simulink model "mavsim_ue"  (R2021b)
settings: Solver=VariableStepAuto  StartTime=0.0  StopTime=48  RelTol=1e-3  EnableMultiTasking=on
InitFcn:
  | param_quad
undefined symbols (not defined in the file or in its folder): P
libraries: slpidlib x4, simulink x1, visionsinks x1, sim3dcameralib x1, sim3dlib x1, uavsim3dlib x1
settings Model: PauseTimes=0.1  Creator=beard  LastModifiedBy=brian
settings SolverCC: ZeroCrossAlgorithm=Adaptive  AlgebraicLoopSolver=TrustRegion
settings DataIOCC: LimitDataPoints=on  SaveFormat=Array  ReturnWorkspaceOutputs=off
settings OptimizationCC: ExpressionDepthLimit=2147483647  InitFltsAndDblsToZero=on  LifeSpan=inf
settings DebuggingCC: UnderspecifiedInitializationDetection=Classic  MergeDetectMultiDrivingBlocksExec=none  IgnoredZcDiagnostic=none  SolverPrmCheckMsg=warning  MultiTaskDSMMsg=warning  MultiTaskCondExecSysMsg=none  StateNameClashWarn=warning  SFUnexpectedBacktrackingDiag=warning  SFNoUnconditionalDefaultTransitionDiag=warning  SFExecutionAtInitializationDiag=none  SFMachineParentedDataDiag=warning  ArithmeticOperatorsInVariantConditions=warning
settings HardwareCC: ProdBitPerPointer=32  ProdBitPerSizeT=32  ProdBitPerPtrDiffT=32  ProdLargestAtomicFloat=None  ProdIntDivRoundTo=Undefined  ProdEndianess=Unspecified  ProdWordSize=32  ProdHWDeviceType=32-bit Generic
settings ModelReferenceCC: PropagateSignalLabelsOutOfModel=off
settings SFSimCC: SimUseLocalCustomCode=off  CustomCodeUndefinedFunction=UseInterfaceOnly
settings RTWCC: RTWUseLocalCustomCode=off
settings CodeAppCC: StateflowObjectComments=on
settings GRTTargetCC: TargetLangStandard=C89/C90 (ANSI)  CombineOutputUpdateFcns=off  GRTInterface=on
settings ConfigComp: CovMetricSettings=dw  CovSaveCumulativeToWorkspaceVar=on  CovSaveSingleToWorkspaceVar=on  CovExternalEMLEnable=off  CovSFcnEnable=off

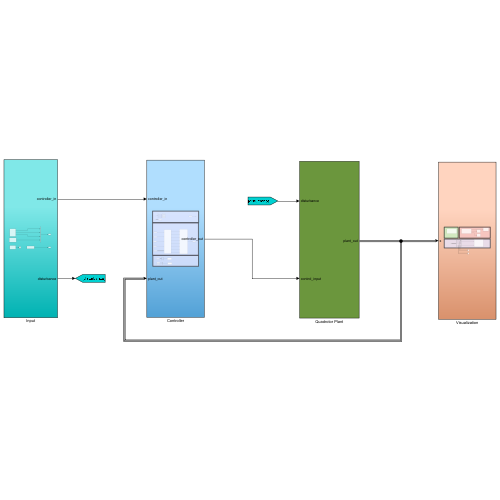
[thumbnail: Simulink's stored preview of the top-level diagram]
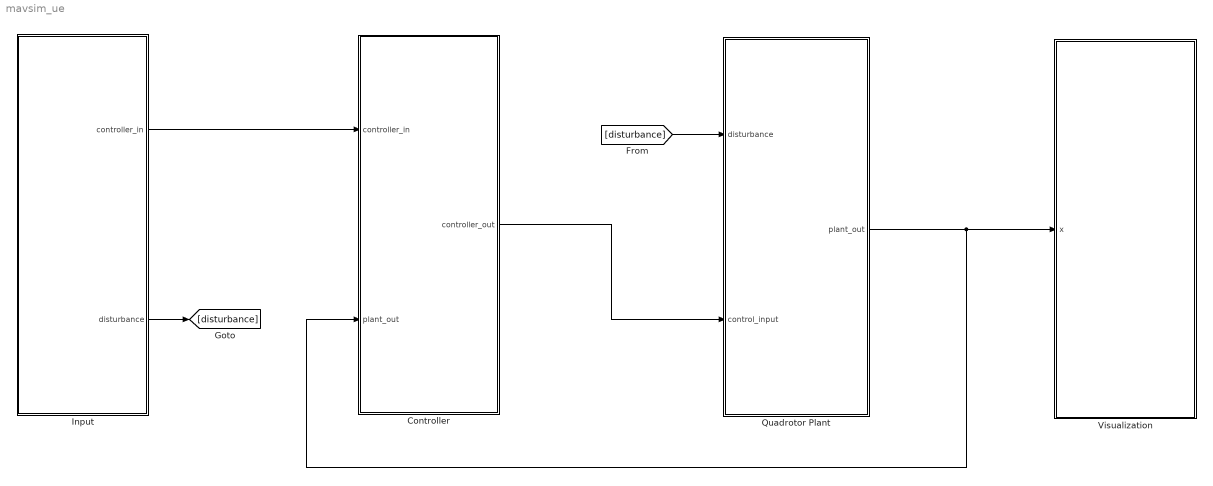
== system mavsim_ue ==
  Controller : Subsystem
  Input : Subsystem
  Quadrotor Plant : Subsystem
  Visualization : Subsystem
  wires:
  Input/2(disturbance) -> [disturbance]
  [disturbance] -> Quadrotor Plant/1(disturbance)
  Quadrotor Plant/1(plant_out) -> Visualization/1(x), Controller/2(plant_out)
  Controller/1(controller_out) -> Quadrotor Plant/2(control_input)
  Input/1(controller_in) -> Controller/1(controller_in)

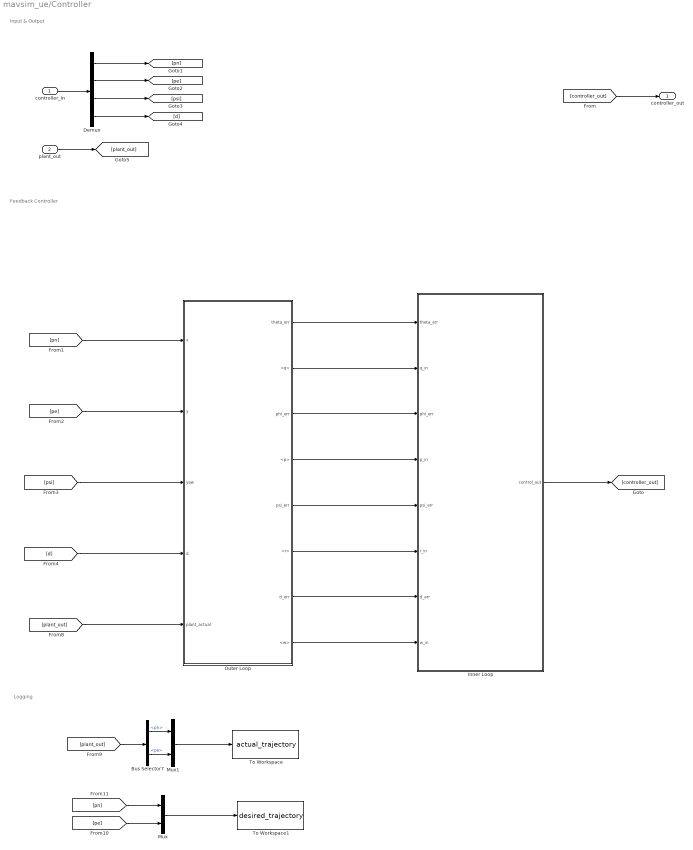
== system mavsim_ue/Controller ==
  note: Logging
  note: Input & Output
  note: Feedback Controller
  controller_in : Inport
  plant_out : Inport  Port=2
  Bus Selector7 : BusSelector  OutputSignals=pn,pe
  Demux : Demux
  Inner Loop : Subsystem
  Mux : Mux  Inputs=2
  Mux1 : Mux  Inputs=2
  Outer Loop : Subsystem
  To Workspace : ToWorkspace  VariableName=actual_trajectory  SaveFormat=Timeseries  SampleTime=-1
  To Workspace1 : ToWorkspace  VariableName=desired_trajectory  SaveFormat=Timeseries  SampleTime=-1
  controller_out : Outport  VectorParamsAs1DForOutWhenUnconnected=off
  wires:
  Inner Loop/1(control_out) -> [controller_out]
  [controller_out] -> controller_out/1
  Demux/1 -> [pn]
  Demux/2 -> [pe]
  Demux/3 -> [psi]
  Demux/4 -> [d]
  plant_out/1 -> [plant_out]
  controller_in/1 -> Demux/1
  [plant_out] -> Bus Selector7/1
  [pe] -> Mux/2
  [pn] -> Mux/1
  Bus Selector7/2 -> Mux1/2  "<pe>"
  Bus Selector7/1 -> Mux1/1  "<pn>"
  Mux1/1 -> To Workspace/1
  Mux/1 -> To Workspace1/1
  [pn] -> Outer Loop/1(x)
  [plant_out] -> Outer Loop/5(plant_actual)
  [pe] -> Outer Loop/2(y)
  [psi] -> Outer Loop/3(yaw)
  [d] -> Outer Loop/4(d)
  Outer Loop/1(theta_err) -> Inner Loop/1(theta_err)
  Outer Loop/2(<q>) -> Inner Loop/2(q_in)
  Outer Loop/3(phi_err) -> Inner Loop/3(phi_err)
  Outer Loop/4(<p>) -> Inner Loop/4(p_in)
  Outer Loop/5(psi_err) -> Inner Loop/5(psi_err)
  Outer Loop/6(<r>) -> Inner Loop/6(r_in)
  Outer Loop/7(d_err) -> Inner Loop/7(d_err)
  Outer Loop/8(<w>) -> Inner Loop/8(w_in)

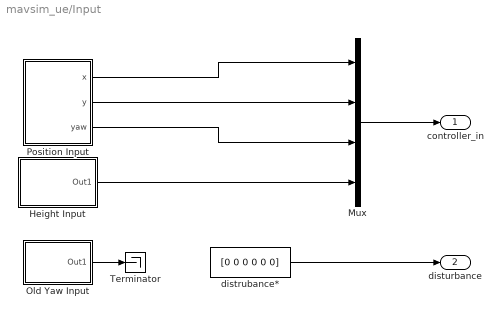
== system mavsim_ue/Input ==
  Height Input : Subsystem
  Mux : Mux
  Old Yaw Input : Subsystem
  Position Input : Subsystem
  Terminator : Terminator
  distrubance* : Constant  Value=[0 0 0 0 0 0]  SampleTime=0
  controller_in : Outport  VectorParamsAs1DForOutWhenUnconnected=off
  disturbance : Outport  Port=2  VectorParamsAs1DForOutWhenUnconnected=off
  wires:
  distrubance*/1 -> disturbance/1
  Mux/1 -> controller_in/1
  Position Input/1(x) -> Mux/1
  Position Input/2(y) -> Mux/2
  Old Yaw Input/1(Out1) -> Terminator/1
  Height Input/1(Out1) -> Mux/4
  Position Input/3(yaw) -> Mux/3

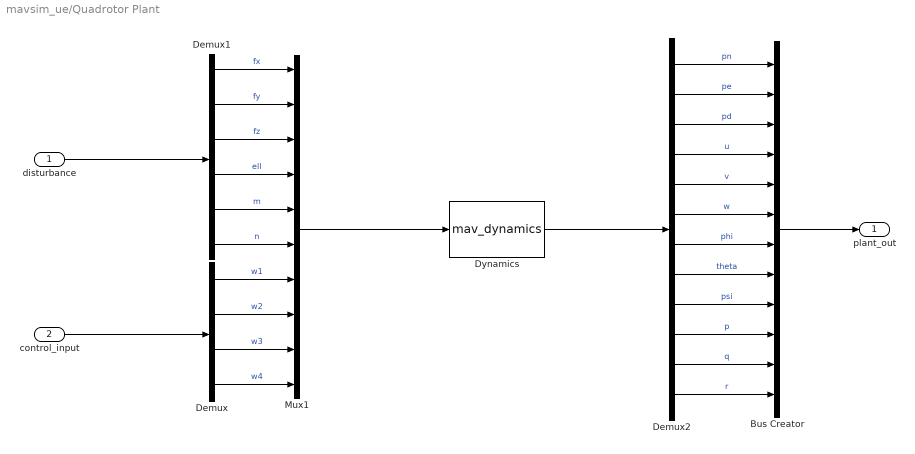
== system mavsim_ue/Quadrotor Plant ==
  disturbance : Inport
  control_input : Inport  Port=2
  Bus Creator : BusCreator  Inputs=12
  Demux : Demux
  Demux1 : Demux  Outputs=6
  Demux2 : Demux  Outputs=12
  Dynamics : S-Function  FunctionName=mav_dynamics  Parameters=P  SFunctionDeploymentMode=off  EnableBusSupport=off
  Mux1 : Mux  Inputs=10
  plant_out : Outport  VectorParamsAs1DForOutWhenUnconnected=off
  wires:
  Dynamics/1 -> Demux2/1
  Demux2/12 -> Bus Creator/12  "r"
  Demux2/1 -> Bus Creator/1  "pn"
  Demux2/2 -> Bus Creator/2  "pe"
  Demux2/3 -> Bus Creator/3  "pd"
  Demux2/4 -> Bus Creator/4  "u"
  Demux2/5 -> Bus Creator/5  "v"
  Demux2/6 -> Bus Creator/6  "w"
  Demux2/8 -> Bus Creator/8  "theta"
  Demux2/7 -> Bus Creator/7  "phi"
  Demux2/9 -> Bus Creator/9  "psi"
  Demux2/10 -> Bus Creator/10  "p"
  Demux2/11 -> Bus Creator/11  "q"
  control_input/1 -> Demux/1
  Bus Creator/1 -> plant_out/1
  Mux1/1 -> Dynamics/1
  Demux/2 -> Mux1/8  "w2"
  Demux1/5 -> Mux1/5  "m"
  Demux1/4 -> Mux1/4  "ell"
  Demux/4 -> Mux1/10  "w4"
  Demux/1 -> Mux1/7  "w1"
  Demux1/6 -> Mux1/6  "n"
  Demux1/2 -> Mux1/2  "fy"
  Demux1/3 -> Mux1/3  "fz"
  Demux/3 -> Mux1/9  "w3"
  Demux1/1 -> Mux1/1  "fx"
  disturbance/1 -> Demux1/1

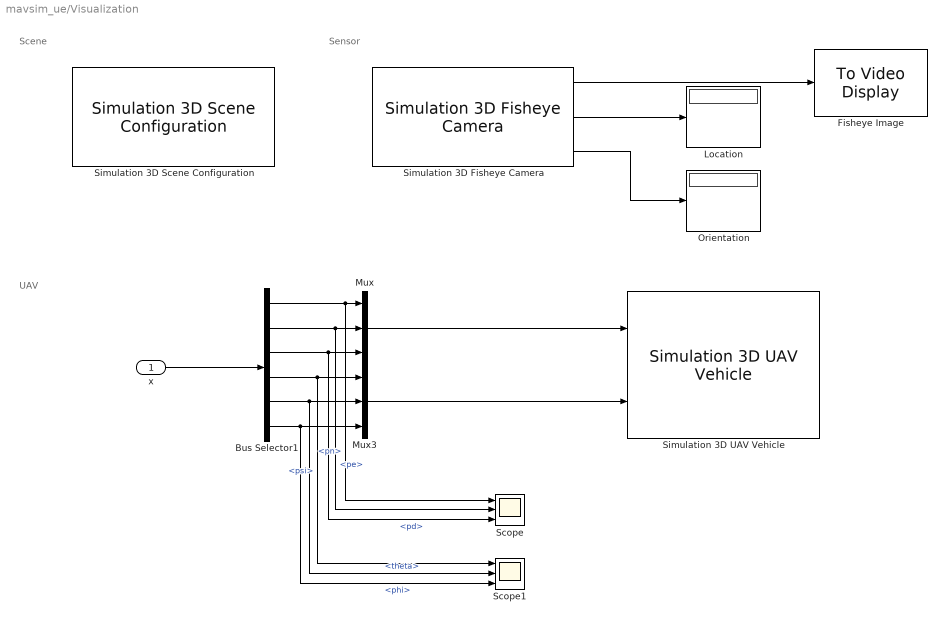
== system mavsim_ue/Visualization ==
  note: Sensor
  note: UAV
  note: Scene
  x : Inport
  Bus Selector1 : BusSelector  OutputSignals=pn,pe,pd,psi,theta,phi
  Fisheye Image : visionsinks/To Video Display  windowSizeMode=Normal  openAtMdlStart=on  fullScreen=off  videoWindowX=3199  videoWindowY=680  saveWindowSize=off  videoWindowWidth=640  videoWindowHeight=502  inputColorFormat=RGB  inputType=Obsolete  imagePorts=One multidimensional signal  OutputDevice=On-screen video monitor  dataOrg=Column-major  isWindowOpen=off
  Location : Display
  Mux : Mux  Inputs=3
  Mux3 : Mux  Inputs=3
  Orientation : Display
  Scope : Scope  NumInputPorts=3
  Scope1 : Scope  NumInputPorts=3
  Simulation 3D Fisheye Camera : sim3dcameralib/Simulation 3D Fisheye Camera  Priority=1  sensorTag=Sim3dSensor2  sensorId=2  sensorName=Sim3dSensor2  vehTagList={'Scene Origin';'SimulinkVehicle2'}  vehTag=SimulinkVehicle2  mountLoc=Origin  offsetFlag=on  tmountOffset=[0.1, 0, 0]  extTmount=off  rmountOffset=[0, 0, 0]  extRmount=off  OpticalCenter=[640, 360]  ImageSize=[720, 1280]  RadialDistortion=[320, -0.0005, 0, 0]  StretchMatrix=[1, 0; 0, 1]  TransformOutportEnabled=on  SampleTime=-1  mountPoint=[0.1 0 0]  mountOrientation=[0 0 0]  aMode=4  ID=2
      settings: SourceProductBaseCode=AE,DR,UV,VE
  Simulation 3D Scene Configuration : sim3dlib/Simulation 3D Scene Configuration  Priority=0  ProjectFormat_internal=Default Scenes  ProjectFormat=Default Scenes  SceneDesc=US city block  ProjectName=C:\Program Files\MATLAB\R2021b\toolbox\shared\sim3d_projects\automotive_project\UE4\WindowsNoEditor\VehicleSimulation.exe  ScenePath=/Game/Maps/USCityBlock  vehTagList={'Scene Origin';'SimulinkVehicle2'}  vehTag=SimulinkVehicle2  OpVisEn=off  Ts=1/60  EnableWindow=on  EnableWeather=off  SunAltitude=40.0  SunAzimuth=90  clouds=10  wind=1  fog=0  rain=0  sensorTag=MainCamera2  sensorId=2  sensorName=MainCamera2  mountLoc=Origin  offsetFlag=off  tmountOffset=[0, 0, 0]  rmountOffset=[0, 0, 0]  HorizontalResolution=1280  VerticalResolution=720  HorizontalFOV=60  mountPoint=[0 0 0]  mountOrientation=[0 0 0]  aMode=4  ID=2
      settings: SourceProductBaseCode=AE,DR,UV,VE
  Simulation 3D UAV Vehicle : uavsim3dlib/Simulation 3D UAV Vehicle  Mesh=Quadrotor  MeshPath=/MathWorksUAVContent/UAVs/HexaRotorUAV/HexaRotor.HexaRotor  Color=Orange  ActorName=SimulinkVehicle2  InitialTranslation=[0 5 1.5]  InitialRotation=[0 0 0]  SampleTime=-1  ActorType=SimulinkVehicle  ID=2  aMode=4  ActorTag=SimulinkVehicle2
      settings: SourceProductBaseCode=UV
  wires:
  Bus Selector1/2 -> Scope/2, Mux/2  "<pe>"
  Simulation 3D Fisheye Camera/3 -> Orientation/1
  Bus Selector1/6 -> Scope1/3, Mux3/3  "<phi>"
  Simulation 3D Fisheye Camera/1 -> Fisheye Image/1
  Bus Selector1/5 -> Scope1/2, Mux3/2  "<theta>"
  Simulation 3D Fisheye Camera/2 -> Location/1
  x/1 -> Bus Selector1/1
  Mux3/1 -> Simulation 3D UAV Vehicle/2
  Mux/1 -> Simulation 3D UAV Vehicle/1
  Bus Selector1/1 -> Scope/1, Mux/1  "<pn>"
  Bus Selector1/3 -> Scope/3, Mux/3  "<pd>"
  Bus Selector1/4 -> Scope1/1, Mux3/1  "<psi>"

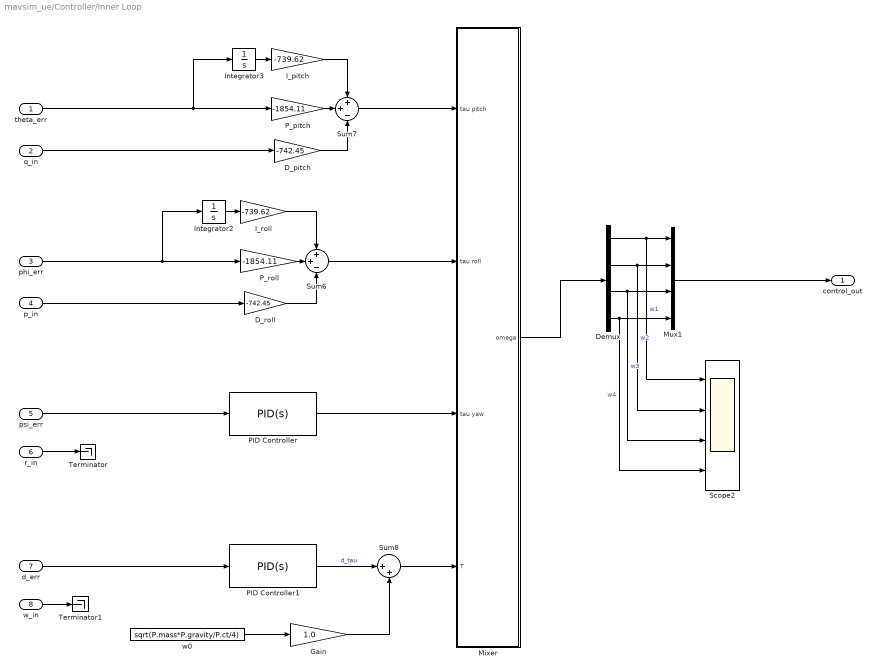
== system mavsim_ue/Controller/Inner Loop ==
  theta_err : Inport
  q_in : Inport  Port=2
  phi_err : Inport  Port=3
  p_in : Inport  Port=4
  psi_err : Inport  Port=5
  r_in : Inport  Port=6
  d_err : Inport  Port=7
  w_in : Inport  Port=8
  D_pitch : Gain  Gain=-742.45
  D_roll : Gain  Gain=-742.45
  Demux : Demux
  Gain : Gain  Gain=1.0
  I_pitch : Gain  Gain=-739.62
  I_roll : Gain  Gain=-739.62
  Integrator2 : Integrator
  Integrator3 : Integrator
  Mixer : Subsystem
  Mux1 : Mux
  PID Controller : slpidlib/PID Controller  Controller=PID  Form=Parallel  TimeDomain=Continuous-time  UseExternalTs=off  SampleTime=1  IntegratorMethod=Forward Euler  FilterMethod=Forward Euler  ControllerParametersSource=internal  P=-13367.2156192971  I=-5976.18350297239  D=-7341.77839074489  UseFilter=on  N=52.0850115715791  TunerSelectOption=Transfer Function Based (PID Tuner App)  InitialConditionSource=internal  InitialConditionForIntegrator=0  InitialConditionForFilter=0  DifferentiatorICPrevScaledInput=0  ExternalReset=none  TrackingMode=off  Kt=1  LimitOutput=off  SatLimitsSource=internal  UpperSaturationLimit=pi/3  LowerSaturationLimit=-pi/3  LinearizeAsGain=off  AntiWindupMode=clamping  Kb=1.5  POutMin=[]  POutMax=[]  IOutMin=[]  IOutMax=[]  DOutMin=[]  DOutMax=[]  NOutMin=[]  NOutMax=[]  SumOutMin=[]  SumOutMax=[]  SaturationOutMin=[]  SaturationOutMax=[]  PParamMin=[]  PParamMax=[]  IParamMin=[]  IParamMax=[]  DParamMin=[]  DParamMax=[]  NParamMin=[]  NParamMax=[]  KbParamMin=[]  KbParamMax=[]  KtParamMin=[]  KtParamMax=[]  KbOutMin=[]  KbOutMax=[]  KtOutMin=[]  KtOutMax=[]  IntegratorOutMin=[]  IntegratorOutMax=[]  FilterOutMin=[]  FilterOutMax=[]  SumI1OutMin=[]  SumI1OutMax=[]  SumI2OutMin=[]  SumI2OutMax=[]  SumI3OutMin=[]  SumI3OutMax=[]  SumI4OutMin=[]  SumI4OutMax=[]  SumDOutMin=[]  SumDOutMax=[]  DifferentiatorOutMin=[]  DifferentiatorOutMax=[]  FilterDiffOutCoefMin=[]  FilterDiffOutCoefMax=[]  ReciprocalOutMin=[]  ReciprocalOutMax=[]  SumDenOutMin=[]  SumDenOutMax=[]  SumNumOutMin=[]  SumNumOutMax=[]  DivideOutMin=[]  DivideOutMax=[]  UdiffTsProdOutMin=[]  UdiffTsProdOutMax=[]  NTsProdOutMin=[]  NTsProdOutMax=[]  UintegralTsProdOutMin=[]  UintegralTsProdOutMax=[]  UngainTsProdOutMin=[]  UngainTsProdOutMax=[]  IntegratorContinuousStateAttributes=''  IntegratorStateMustResolveToSignalObject=off  IntegratorRTWStateStorageClass=Auto  FilterContinuousStateAttributes=''  FilterStateMustResolveToSignalObject=off  FilterRTWStateStorageClass=Auto  ParallelPVariant=InternalParameters  IdealPVariant=Disabled  IVariant=InternalParameters  DVariant=InternalParameters  IntegratorVariant=Continuous  SatVariant=Disabled  AWVariant=Passthrough  PCopyVariant=Disabled  TRVariant=Disabled  FdbkBlocksVariant=Forward  IdealPFdbkVariant=Disabled  SatFdbkVariant=Disabled  DerivativeFilterVariant=ContFilter  NVariant=InternalParameters  NCopyVariant=Disabled  FilterICVariant=InternalICsFilter  IntegratorICVariant=InternalICs  ExternalResetVariant=Disabled  TRSumVariant=Passthrough  SumFdbkVariant=Disabled  SumVariant=Sum_PID  TsampFilterVariant=InternalTs  TsampNgainVariant=Passthrough  TsampIntegralVariant=Passthrough  ExternalSaturationOutDataTypeStr=Inherit: Same as second input
  PID Controller1 : slpidlib/PID Controller  Controller=PID  Form=Parallel  TimeDomain=Continuous-time  UseExternalTs=off  SampleTime=1  IntegratorMethod=Forward Euler  FilterMethod=Forward Euler  ControllerParametersSource=internal  P=949.514869239601  I=444.513280768002  D=498.037549912903  UseFilter=on  N=54.5397025421619  TunerSelectOption=Transfer Function Based (PID Tuner App)  InitialConditionSource=internal  InitialConditionForIntegrator=0  InitialConditionForFilter=0  DifferentiatorICPrevScaledInput=0  ExternalReset=none  TrackingMode=off  Kt=1  LimitOutput=off  SatLimitsSource=internal  UpperSaturationLimit=pi/3  LowerSaturationLimit=-pi/3  LinearizeAsGain=off  AntiWindupMode=clamping  Kb=1.5  POutMin=[]  POutMax=[]  IOutMin=[]  IOutMax=[]  DOutMin=[]  DOutMax=[]  NOutMin=[]  NOutMax=[]  SumOutMin=[]  SumOutMax=[]  SaturationOutMin=[]  SaturationOutMax=[]  PParamMin=[]  PParamMax=[]  IParamMin=[]  IParamMax=[]  DParamMin=[]  DParamMax=[]  NParamMin=[]  NParamMax=[]  KbParamMin=[]  KbParamMax=[]  KtParamMin=[]  KtParamMax=[]  KbOutMin=[]  KbOutMax=[]  KtOutMin=[]  KtOutMax=[]  IntegratorOutMin=[]  IntegratorOutMax=[]  FilterOutMin=[]  FilterOutMax=[]  SumI1OutMin=[]  SumI1OutMax=[]  SumI2OutMin=[]  SumI2OutMax=[]  SumI3OutMin=[]  SumI3OutMax=[]  SumI4OutMin=[]  SumI4OutMax=[]  SumDOutMin=[]  SumDOutMax=[]  DifferentiatorOutMin=[]  DifferentiatorOutMax=[]  FilterDiffOutCoefMin=[]  FilterDiffOutCoefMax=[]  ReciprocalOutMin=[]  ReciprocalOutMax=[]  SumDenOutMin=[]  SumDenOutMax=[]  SumNumOutMin=[]  SumNumOutMax=[]  DivideOutMin=[]  DivideOutMax=[]  UdiffTsProdOutMin=[]  UdiffTsProdOutMax=[]  NTsProdOutMin=[]  NTsProdOutMax=[]  UintegralTsProdOutMin=[]  UintegralTsProdOutMax=[]  UngainTsProdOutMin=[]  UngainTsProdOutMax=[]  IntegratorContinuousStateAttributes=''  IntegratorStateMustResolveToSignalObject=off  IntegratorRTWStateStorageClass=Auto  FilterContinuousStateAttributes=''  FilterStateMustResolveToSignalObject=off  FilterRTWStateStorageClass=Auto  ParallelPVariant=InternalParameters  IdealPVariant=Disabled  IVariant=InternalParameters  DVariant=InternalParameters  IntegratorVariant=Continuous  SatVariant=Disabled  AWVariant=Passthrough  PCopyVariant=Disabled  TRVariant=Disabled  FdbkBlocksVariant=Forward  IdealPFdbkVariant=Disabled  SatFdbkVariant=Disabled  DerivativeFilterVariant=ContFilter  NVariant=InternalParameters  NCopyVariant=Disabled  FilterICVariant=InternalICsFilter  IntegratorICVariant=InternalICs  ExternalResetVariant=Disabled  TRSumVariant=Passthrough  SumFdbkVariant=Disabled  SumVariant=Sum_PID  TsampFilterVariant=InternalTs  TsampNgainVariant=Passthrough  TsampIntegralVariant=Passthrough  ExternalSaturationOutDataTypeStr=Inherit: Same as second input
  P_pitch : Gain  Gain=-1854.11
  P_roll : Gain  Gain=-1854.11
  Scope2 : Scope  NumInputPorts=4
  Sum6 : Sum  Inputs=++-
  Sum7 : Sum  Inputs=++-
  Sum8 : Sum  Inputs=|++
  Terminator : Terminator
  Terminator1 : Terminator
  w0 : Constant  Value=sqrt(P.mass*P.gravity/P.ct/4)  SampleTime=0
  control_out : Outport  VectorParamsAs1DForOutWhenUnconnected=off
  wires:
  r_in/1 -> Terminator/1
  P_pitch/1 -> Sum7/2
  P_roll/1 -> Sum6/2
  Demux/4 -> Mux1/4, Scope2/4  "w4"
  Demux/1 -> Mux1/1, Scope2/1  "w1"
  theta_err/1 -> Integrator3/1, P_pitch/1
  Demux/2 -> Mux1/2, Scope2/2  "w2"
  Sum8/1 -> Mixer/4(T)
  Mixer/1(omega) -> Demux/1
  phi_err/1 -> Integrator2/1, P_roll/1
  D_roll/1 -> Sum6/3
  Integrator2/1 -> I_roll/1
  Integrator3/1 -> I_pitch/1
  D_pitch/1 -> Sum7/3
  Demux/3 -> Mux1/3, Scope2/3  "w3"
  I_pitch/1 -> Sum7/1
  q_in/1 -> D_pitch/1
  w0/1 -> Gain/1
  I_roll/1 -> Sum6/1
  Mux1/1 -> control_out/1
  Sum6/1 -> Mixer/2(tau roll)
  w_in/1 -> Terminator1/1
  Sum7/1 -> Mixer/1(tau pitch)
  p_in/1 -> D_roll/1
  psi_err/1 -> PID Controller/1
  PID Controller/1 -> Mixer/3(tau yaw)
  PID Controller1/1 -> Sum8/1  "d_tau"
  d_err/1 -> PID Controller1/1
  Gain/1 -> Sum8/2

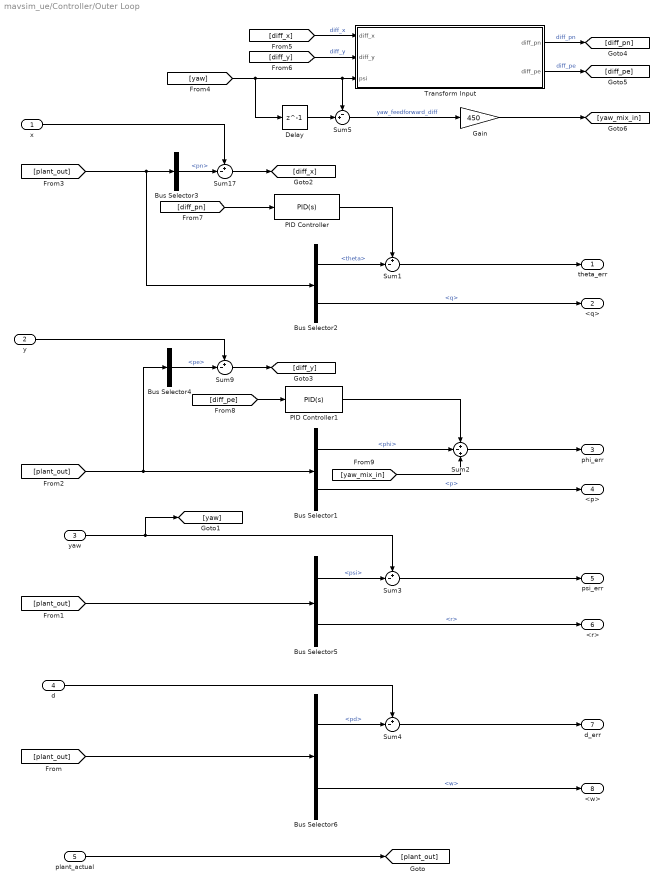
== system mavsim_ue/Controller/Outer Loop ==
  x : Inport
  y : Inport  Port=2
  yaw : Inport  Port=3
  d : Inport  Port=4
  plant_actual : Inport  Port=5
  Bus Selector1 : BusSelector  OutputSignals=phi,p
  Bus Selector2 : BusSelector  OutputSignals=theta,q
  Bus Selector3 : BusSelector  OutputSignals=pn
  Bus Selector4 : BusSelector  OutputSignals=pe
  Bus Selector5 : BusSelector  OutputSignals=psi,r
  Bus Selector6 : BusSelector  OutputSignals=pd,w
  Delay : Delay  DelayLength=1
  Gain : Gain  Gain=450
  PID Controller : slpidlib/PID Controller  Controller=PID  Form=Parallel  TimeDomain=Continuous-time  UseExternalTs=off  SampleTime=1  IntegratorMethod=Forward Euler  FilterMethod=Forward Euler  ControllerParametersSource=internal  P=0.00699656063641612  I=6.00915879281628e-05  D=0.106583930326049  UseFilter=on  N=132.721128235741  TunerSelectOption=Transfer Function Based (PID Tuner App)  InitialConditionSource=internal  InitialConditionForIntegrator=0  InitialConditionForFilter=0  DifferentiatorICPrevScaledInput=0  ExternalReset=none  TrackingMode=off  Kt=0.1  LimitOutput=on  SatLimitsSource=internal  UpperSaturationLimit=pi/2.2  LowerSaturationLimit=-pi/2.2  LinearizeAsGain=off  AntiWindupMode=clamping  Kb=1.5  POutMin=[]  POutMax=[]  IOutMin=[]  IOutMax=[]  DOutMin=[]  DOutMax=[]  NOutMin=[]  NOutMax=[]  SumOutMin=[]  SumOutMax=[]  SaturationOutMin=[]  SaturationOutMax=[]  PParamMin=[]  PParamMax=[]  IParamMin=[]  IParamMax=[]  DParamMin=[]  DParamMax=[]  NParamMin=[]  NParamMax=[]  KbParamMin=[]  KbParamMax=[]  KtParamMin=[]  KtParamMax=[]  KbOutMin=[]  KbOutMax=[]  KtOutMin=[]  KtOutMax=[]  IntegratorOutMin=[]  IntegratorOutMax=[]  FilterOutMin=[]  FilterOutMax=[]  SumI1OutMin=[]  SumI1OutMax=[]  SumI2OutMin=[]  SumI2OutMax=[]  SumI3OutMin=[]  SumI3OutMax=[]  SumI4OutMin=[]  SumI4OutMax=[]  SumDOutMin=[]  SumDOutMax=[]  DifferentiatorOutMin=[]  DifferentiatorOutMax=[]  FilterDiffOutCoefMin=[]  FilterDiffOutCoefMax=[]  ReciprocalOutMin=[]  ReciprocalOutMax=[]  SumDenOutMin=[]  SumDenOutMax=[]  SumNumOutMin=[]  SumNumOutMax=[]  DivideOutMin=[]  DivideOutMax=[]  UdiffTsProdOutMin=[]  UdiffTsProdOutMax=[]  NTsProdOutMin=[]  NTsProdOutMax=[]  UintegralTsProdOutMin=[]  UintegralTsProdOutMax=[]  UngainTsProdOutMin=[]  UngainTsProdOutMax=[]  IntegratorContinuousStateAttributes=''  IntegratorStateMustResolveToSignalObject=off  IntegratorRTWStateStorageClass=Auto  FilterContinuousStateAttributes=''  FilterStateMustResolveToSignalObject=off  FilterRTWStateStorageClass=Auto  ParallelPVariant=InternalParameters  IdealPVariant=Disabled  IVariant=InternalParameters  DVariant=InternalParameters  IntegratorVariant=Continuous  SatVariant=Enabled  AWVariant=ContClampingParallel  PCopyVariant=Disabled  TRVariant=Disabled  FdbkBlocksVariant=Forward  IdealPFdbkVariant=Disabled  SatFdbkVariant=Disabled  DerivativeFilterVariant=ContFilter  NVariant=InternalParameters  NCopyVariant=Disabled  FilterICVariant=InternalICsFilter  IntegratorICVariant=InternalICs  ExternalResetVariant=Disabled  TRSumVariant=Passthrough  SumFdbkVariant=Disabled  SumVariant=Sum_PID  TsampFilterVariant=InternalTs  TsampNgainVariant=Passthrough  TsampIntegralVariant=Passthrough  ExternalSaturationOutDataTypeStr=Inherit: Same as second input
  PID Controller1 : slpidlib/PID Controller  Controller=PID  Form=Parallel  TimeDomain=Continuous-time  UseExternalTs=off  SampleTime=1  IntegratorMethod=Forward Euler  FilterMethod=Forward Euler  ControllerParametersSource=internal  P=-0.0043801368418265  I=-3.38745804747184e-05  D=-0.112019721849609  UseFilter=on  N=138.65464157868  TunerSelectOption=Transfer Function Based (PID Tuner App)  InitialConditionSource=internal  InitialConditionForIntegrator=0  InitialConditionForFilter=0  DifferentiatorICPrevScaledInput=0  ExternalReset=none  TrackingMode=off  Kt=0.75  LimitOutput=on  SatLimitsSource=internal  UpperSaturationLimit=pi/2.2  LowerSaturationLimit=-pi/2.2  LinearizeAsGain=off  AntiWindupMode=clamping  Kb=1  POutMin=[]  POutMax=[]  IOutMin=[]  IOutMax=[]  DOutMin=[]  DOutMax=[]  NOutMin=[]  NOutMax=[]  SumOutMin=[]  SumOutMax=[]  SaturationOutMin=[]  SaturationOutMax=[]  PParamMin=[]  PParamMax=[]  IParamMin=[]  IParamMax=[]  DParamMin=[]  DParamMax=[]  NParamMin=[]  NParamMax=[]  KbParamMin=[]  KbParamMax=[]  KtParamMin=[]  KtParamMax=[]  KbOutMin=[]  KbOutMax=[]  KtOutMin=[]  KtOutMax=[]  IntegratorOutMin=[]  IntegratorOutMax=[]  FilterOutMin=[]  FilterOutMax=[]  SumI1OutMin=[]  SumI1OutMax=[]  SumI2OutMin=[]  SumI2OutMax=[]  SumI3OutMin=[]  SumI3OutMax=[]  SumI4OutMin=[]  SumI4OutMax=[]  SumDOutMin=[]  SumDOutMax=[]  DifferentiatorOutMin=[]  DifferentiatorOutMax=[]  FilterDiffOutCoefMin=[]  FilterDiffOutCoefMax=[]  ReciprocalOutMin=[]  ReciprocalOutMax=[]  SumDenOutMin=[]  SumDenOutMax=[]  SumNumOutMin=[]  SumNumOutMax=[]  DivideOutMin=[]  DivideOutMax=[]  UdiffTsProdOutMin=[]  UdiffTsProdOutMax=[]  NTsProdOutMin=[]  NTsProdOutMax=[]  UintegralTsProdOutMin=[]  UintegralTsProdOutMax=[]  UngainTsProdOutMin=[]  UngainTsProdOutMax=[]  IntegratorContinuousStateAttributes=''  IntegratorStateMustResolveToSignalObject=off  IntegratorRTWStateStorageClass=Auto  FilterContinuousStateAttributes=''  FilterStateMustResolveToSignalObject=off  FilterRTWStateStorageClass=Auto  ParallelPVariant=InternalParameters  IdealPVariant=Disabled  IVariant=InternalParameters  DVariant=InternalParameters  IntegratorVariant=Continuous  SatVariant=Enabled  AWVariant=ContClampingParallel  PCopyVariant=Disabled  TRVariant=Disabled  FdbkBlocksVariant=Forward  IdealPFdbkVariant=Disabled  SatFdbkVariant=Disabled  DerivativeFilterVariant=ContFilter  NVariant=InternalParameters  NCopyVariant=Disabled  FilterICVariant=InternalICsFilter  IntegratorICVariant=InternalICs  ExternalResetVariant=Disabled  TRSumVariant=Passthrough  SumFdbkVariant=Disabled  SumVariant=Sum_PID  TsampFilterVariant=InternalTs  TsampNgainVariant=Passthrough  TsampIntegralVariant=Passthrough  ExternalSaturationOutDataTypeStr=Inherit: Same as second input
  Sum{1,3..4,9,17} (5 alike) : Sum  Inputs=+-|
  Sum2 : Sum  Inputs=+-+
  Sum5 : Sum  Inputs=-+|
  Transform Input : MATLAB Function  TreatAsAtomicUnit=on
  theta_err : Outport
  <q> : Outport  Port=2
  phi_err : Outport  Port=3
  <p> : Outport  Port=4
  psi_err : Outport  Port=5
  <r> : Outport  Port=6
  d_err : Outport  Port=7
  <w> : Outport  Port=8
  wires:
  [plant_out] -> Bus Selector2/1, Bus Selector3/1
  Bus Selector4/1 -> Sum9/2  "<pe>"
  Bus Selector2/1 -> Sum1/2  "<theta>"
  Bus Selector6/2 -> <w>/1  "<w>"
  Bus Selector1/1 -> Sum2/2  "<phi>"
  Bus Selector3/1 -> Sum17/2  "<pn>"
  Bus Selector5/1 -> Sum3/2  "<psi>"
  Bus Selector6/1 -> Sum4/2  "<pd>"
  [plant_out] -> Bus Selector5/1
  Bus Selector2/2 -> <q>/1  "<q>"
  [plant_out] -> Bus Selector4/1, Bus Selector1/1
  Sum9/1 -> [diff_y]
  [plant_out] -> Bus Selector6/1
  yaw/1 -> [yaw], Sum3/1
  x/1 -> Sum17/1
  Sum3/1 -> psi_err/1
  y/1 -> Sum9/1
  Bus Selector5/2 -> <r>/1  "<r>"
  Bus Selector1/2 -> <p>/1  "<p>"
  plant_actual/1 -> [plant_out]
  Sum4/1 -> d_err/1
  d/1 -> Sum4/1
  Sum17/1 -> [diff_x]
  Sum1/1 -> theta_err/1
  Sum2/1 -> phi_err/1
  [yaw] -> Delay/1, Transform Input/3(psi), Sum5/1
  [diff_x] -> Transform Input/1(diff_x)  "diff_x"
  [diff_y] -> Transform Input/2(diff_y)  "diff_y"
  Transform Input/1(diff_pn) -> [diff_pn]  "diff_pn"
  [diff_pn] -> PID Controller/1
  [diff_pe] -> PID Controller1/1
  Delay/1 -> Sum5/2
  Sum5/1 -> Gain/1  "yaw_feedforward_diff"
  Transform Input/2(diff_pe) -> [diff_pe]  "diff_pe"
  Gain/1 -> [yaw_mix_in]
  [yaw_mix_in] -> Sum2/3
  PID Controller/1 -> Sum1/1
  PID Controller1/1 -> Sum2/1

== system mavsim_ue/Input/Height Input ==
  Constant : Constant  Value=0
  Manual Switch3 : ManualSwitch  CurrentSetting=0
  Takeoff : Subsystem
  Out1 : Outport
  wires:
  Constant/1 -> Manual Switch3/1
  Manual Switch3/1 -> Out1/1
  Takeoff/1(x) -> Manual Switch3/2

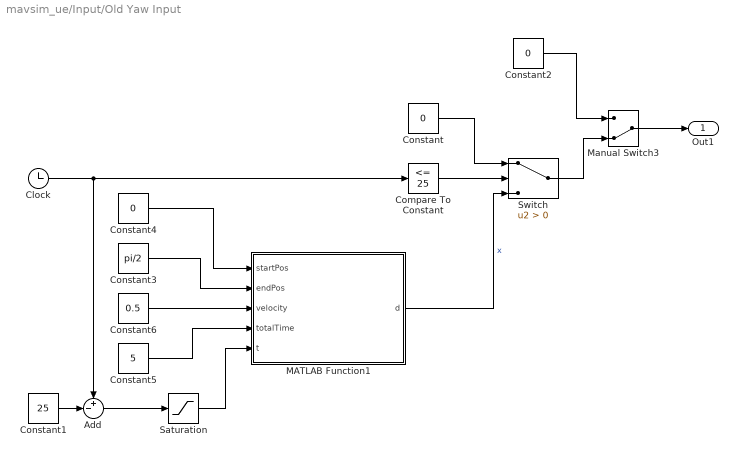
== system mavsim_ue/Input/Old Yaw Input ==
  Add : Sum  Inputs=+-|
  Clock : Clock
  Compare To Constant : simulink/Logic and Bit Operations/Compare To Constant  relop=<=  const=25  OutDataTypeStr=boolean
  Constant : Constant  Value=0
  Constant1 : Constant  Value=25
  Constant2 : Constant  Value=0
  Constant3 : Constant  Value=pi/2
  Constant4 : Constant  Value=0
  Constant5 : Constant  Value=5
  Constant6 : Constant  Value=0.5
  MATLAB Function1 : MATLAB Function  TreatAsAtomicUnit=on  SystemSampleTime=0.001
  Manual Switch3 : ManualSwitch  CurrentSetting=0
  Saturation : Saturate  UpperLimit=250  LowerLimit=0
  Switch : Switch  Criteria=u2 > Threshold
  Out1 : Outport
  wires:
  Constant/1 -> Switch/1
  Clock/1 -> Compare To Constant/1, Add/1
  Compare To Constant/1 -> Switch/2
  Constant4/1 -> MATLAB Function1/1(startPos)
  MATLAB Function1/1(d) -> Switch/3  "x"
  Add/1 -> Saturation/1
  Constant5/1 -> MATLAB Function1/4(totalTime)
  Constant3/1 -> MATLAB Function1/2(endPos)
  Constant6/1 -> MATLAB Function1/3(velocity)
  Constant1/1 -> Add/2
  Saturation/1 -> MATLAB Function1/5(t)
  Switch/1 -> Manual Switch3/2
  Manual Switch3/1 -> Out1/1
  Constant2/1 -> Manual Switch3/1

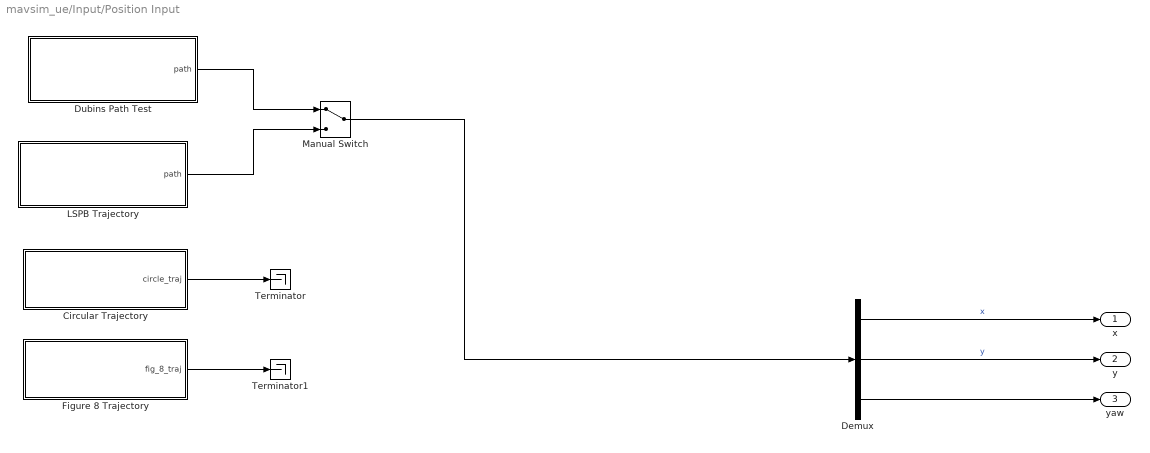
== system mavsim_ue/Input/Position Input ==
  Circular Trajectory : Subsystem
  Demux : Demux  Outputs=3
  Dubins Path Test : Subsystem
  Figure 8 Trajectory : Subsystem
  LSPB Trajectory : Subsystem
  Manual Switch : ManualSwitch
  Terminator : Terminator
  Terminator1 : Terminator
  x : Outport
  y : Outport  Port=2
  yaw : Outport  Port=3
  wires:
  Manual Switch/1 -> Demux/1
  Demux/1 -> x/1  "x"
  Demux/2 -> y/1  "y"
  Circular Trajectory/1(circle_traj) -> Terminator/1
  Figure 8 Trajectory/1(fig_8_traj) -> Terminator1/1
  Demux/3 -> yaw/1
  LSPB Trajectory/1(path) -> Manual Switch/2
  Dubins Path Test/1(path) -> Manual Switch/1

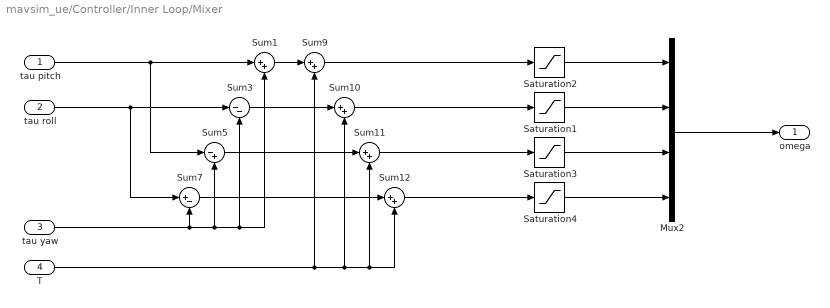
== system mavsim_ue/Controller/Inner Loop/Mixer ==
  tau pitch : Inport
  tau roll : Inport  Port=2
  tau yaw : Inport  Port=3
  T : Inport  Port=4
  Mux2 : Mux
  Saturation{1..4} (4 alike) : Saturate  UpperLimit=20000  LowerLimit=0
  Sum{1,9..12} (5 alike) : Sum  Inputs=|++  InputSameDT=on  SaturateOnIntegerOverflow=on  OutDataTypeStr=Inherit: Same as first input
  Sum3 : Sum  Inputs=|--  InputSameDT=on  SaturateOnIntegerOverflow=on  OutDataTypeStr=Inherit: Same as first input
  Sum5 : Sum  Inputs=|-+  InputSameDT=on  SaturateOnIntegerOverflow=on  OutDataTypeStr=Inherit: Same as first input
  Sum7 : Sum  Inputs=|+-  InputSameDT=on  SaturateOnIntegerOverflow=on  OutDataTypeStr=Inherit: Same as first input
  omega : Outport  VectorParamsAs1DForOutWhenUnconnected=off
  wires:
  Mux2/1 -> omega/1
  tau yaw/1 -> Sum7/2, Sum5/2, Sum3/2, Sum1/2
  Saturation2/1 -> Mux2/1
  Saturation1/1 -> Mux2/2
  Saturation3/1 -> Mux2/3
  Saturation4/1 -> Mux2/4
  tau pitch/1 -> Sum1/1, Sum5/1
  Sum1/1 -> Sum9/1
  Sum3/1 -> Sum10/1
  Sum5/1 -> Sum11/1
  Sum7/1 -> Sum12/1
  Sum9/1 -> Saturation2/1
  Sum10/1 -> Saturation1/1
  Sum11/1 -> Saturation3/1
  Sum12/1 -> Saturation4/1
  T/1 -> Sum11/2, Sum12/2, Sum10/2, Sum9/2
  tau roll/1 -> Sum3/1, Sum7/1

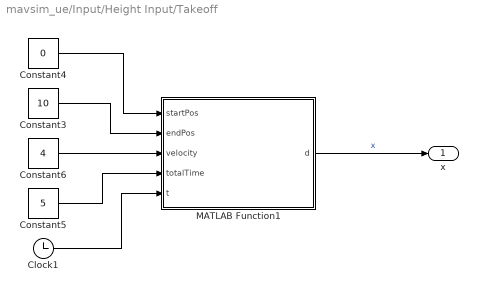
== system mavsim_ue/Input/Height Input/Takeoff ==
  Clock1 : Clock
  Constant3 : Constant  Value=10
  Constant4 : Constant  Value=0
  Constant5 : Constant  Value=5
  Constant6 : Constant  Value=4
  MATLAB Function1 : MATLAB Function  TreatAsAtomicUnit=on  SystemSampleTime=0.001
  x : Outport
  wires:
  Constant3/1 -> MATLAB Function1/2(endPos)
  Constant6/1 -> MATLAB Function1/3(velocity)
  MATLAB Function1/1(d) -> x/1  "x"
  Constant5/1 -> MATLAB Function1/4(totalTime)
  Clock1/1 -> MATLAB Function1/5(t)
  Constant4/1 -> MATLAB Function1/1(startPos)

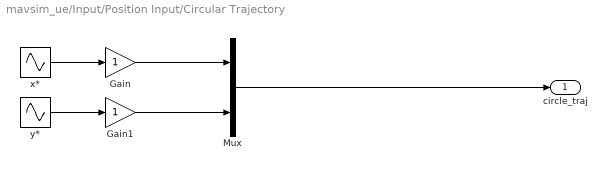
== system mavsim_ue/Input/Position Input/Circular Trajectory ==
  Gain : Gain
  Gain1 : Gain
  Mux : Mux  Inputs=2
  x* : Sin  Amplitude=50  Frequency=2*pi*.1  SampleTime=0
  y* : Sin  Amplitude=50  Frequency=2*pi*.1  Phase=pi/2  SampleTime=0
  circle_traj : Outport  VectorParamsAs1DForOutWhenUnconnected=off
  wires:
  Mux/1 -> circle_traj/1
  Gain1/1 -> Mux/2
  Gain/1 -> Mux/1
  x*/1 -> Gain/1
  y*/1 -> Gain1/1

== system mavsim_ue/Input/Position Input/Dubins Path Test ==
  Clock : Clock
  Constant1 : Constant  Value=2
  Dubins Path : MATLAB Function  TreatAsAtomicUnit=on  SystemSampleTime=0.001
  Mux2 : Mux  Inputs=3
  Scope : Scope  NumInputPorts=3
  path : Outport
  wires:
  Dubins Path/2(y) -> Scope/2, Mux2/2  "y"
  Constant1/1 -> Dubins Path/1(velocity)
  Mux2/1 -> path/1
  Dubins Path/1(x) -> Scope/1, Mux2/1  "x"
  Clock/1 -> Dubins Path/2(t)
  Dubins Path/3(yaw) -> Scope/3, Mux2/3  "yaw"

== system mavsim_ue/Input/Position Input/Figure 8 Trajectory ==
  Gain : Gain  Gain=3
  Gain1 : Gain  Gain=3
  Mux : Mux  Inputs=2
  x* : Sin  Amplitude=50  Frequency=4*pi*.0125  SampleTime=0
  y* : Sin  Amplitude=50  Frequency=2*pi*.0125  SampleTime=0
  fig_8_traj : Outport  VectorParamsAs1DForOutWhenUnconnected=off
  wires:
  Mux/1 -> fig_8_traj/1
  Gain1/1 -> Mux/2
  Gain/1 -> Mux/1
  x*/1 -> Gain/1
  y*/1 -> Gain1/1

== system mavsim_ue/Input/Position Input/LSPB Trajectory ==
  Clock : Clock
  Constant1 : Constant  Value=2
  MATLAB Function2 : MATLAB Function  TreatAsAtomicUnit=on  SystemSampleTime=0.001
  Mux2 : Mux  Inputs=3
  Scope : Scope  NumInputPorts=3
  path : Outport
  wires:
  MATLAB Function2/2(y) -> Scope/2, Mux2/2  "y"
  Constant1/1 -> MATLAB Function2/1(velocity)
  Mux2/1 -> path/1
  MATLAB Function2/1(x) -> Scope/1, Mux2/1  "x"
  Clock/1 -> MATLAB Function2/2(t)
  MATLAB Function2/3(yaw) -> Scope/3, Mux2/3  "yaw"

== matlab function mavsim_ue/Input/Position Input/LSPB Trajectory/MATLAB Function2 ==
  settings: updateMethod=DISCRETE
  data: velocity input; x output; t input; y output; yaw output


function [x, y, yaw] = test_trajectory(velocity, t)
    x = LSPB(0, 76.4, t, velocity*2, 20);
    if (t < 32)
        y = 0;
    else
        yt = t - 32;
        y = LSPB(0, 108, yt, velocity*2, 30);
    end
    if (t<=25)
        yaw = 0;
    else
        yawt = t - 25;
        yaw = LSPB(0,pi/2,yawt,0.5,5.0);
    end
end

== matlab function mavsim_ue/Input/Old Yaw Input/MATLAB Function1 ==
  settings: updateMethod=DISCRETE
  data: startPos input; endPos input; velocity input; totalTime input; d output; t input
function d = test_trajectory(startPos, endPos, velocity, totalTime, t)
d = LSPB(startPos, endPos, t, velocity, totalTime);
end

== matlab function mavsim_ue/Input/Height Input/Takeoff/MATLAB Function1 ==
  settings: updateMethod=DISCRETE
  data: startPos input; endPos input; velocity input; totalTime input; d output; t input
function d = test_trajectory(startPos, endPos, velocity, totalTime, t)
d = LSPB(startPos, endPos, t, velocity, totalTime);
end

== matlab function mavsim_ue/Controller/Outer Loop/Transform Input ==
  data: diff_x input; diff_pn output; diff_y input; psi input; diff_pe output
function [ diff_pn,  diff_pe] = fcn(diff_x, diff_y, psi)

% diff_pn = diff_x*cos(psi) + diff_y*cos(pi/2 - psi);
% diff_pe = -diff_x*sin(pi/2 - psi) - diff_y*sin(pi/2 - psi);

diff_pn = diff_x*sin(pi/2 - psi) + diff_y*cos(pi/2 - psi);
diff_pe = -diff_x*cos(pi/2 - psi) + diff_y*sin(pi/2 - psi);

== matlab function mavsim_ue/Input/Position Input/Dubins Path Test/Dubins Path ==
  settings: updateMethod=DISCRETE
  data: velocity input; x output; t input; y output; yaw output


function [x, y, yaw] = dubins_path(velocity, t)
    persistent time_offset1 time_offset2 radius turn_time
    if isempty(time_offset2)
        time_offset1 = 20;
        time_offset2 = 24;
        radius = 24.0;
        turn_time = 10.0;
    end

    if (t < time_offset1)
        x = LSPB(0, 76.4, t, velocity*2, 20);
        y = 0;
        yaw = 0;
        if (x >= (76.4-radius))
            time_offset1 = t;
            time_offset2 = time_offset1 + turn_time;
        end
    elseif (t < time_offset2)
        theta = ((pi/2) / (time_offset2 - time_offset1)) * (t-time_offset1);
        x = radius*sin(theta) - radius + 76.4;
        y = radius - radius*cos(theta);
        yaw = theta;
    else
        yt = t-time_offset2+7.5;
        x = 76.4;
        y = LSPB(0, 108, yt, velocity*2, 30);
        yaw = pi/2;
    end
end
